simulink model "ammclib_gflib_pip_s32k14x"  (Simulink 9.0)
settings: Solver=FixedStepDiscrete  StartTime=0.0  StopTime=5  FixedStep=0.001  RelTol=1e-3  EnableMultiTasking=on
InitFcn:
  | mbd_s32k_consistency_checks(bdroot(gcs));
undefined symbols (not defined in the file or in its folder): LQFP
libraries: ammclib_bam_s32k14x x12, mbd_s32k1xx_ec_toolbox x2, simulink x1
Description:
  | This model tests the AMMCLIB GFLIB PI Parallel Form Controller blocks
  | 
  | Validation:
  | - Run the model in Simulation and check if the results look like the ones shown in the scope capture
  | - Open Freemaster (ammclib_gflib_pip_s32k14x.pmp) and compare the HW results against the Simulated ones
CloseFcn:
  | clear all;
settings Model: Creator=NXP MBDT Team  LastModifiedBy=nxf35172
settings DataIOCC: ExternalInput=off  InitialState=off  LimitDataPoints=on  SaveOutput=off  SignalLogging=off  SaveTime=off
settings OptimizationCC: DefaultParameterBehavior=Inlined  LifeSpan=1
settings DebuggingCC: SolverPrmCheckMsg=warning  InheritedTsInSrcMsg=none  SingleTaskRateTransMsg=error  ParameterPrecisionLossMsg=none  UnconnectedInputMsg=error  UnconnectedOutputMsg=error  UnconnectedLineMsg=error  AllowSymbolicDim=off  UnknownTsInhSupMsg=error  StateNameClashWarn=warning
settings HardwareCC: ProdLargestAtomicInteger=Long  ProdLargestAtomicFloat=Double  ProdEndianess=LittleEndian  ProdHWDeviceType=ARM Compatible->ARM Cortex
settings SFSimCC: MATLABDynamicMemAlloc=off
settings RTWCC: SystemTargetFile=mbd_s32k.tlc  MakeCommand=mbd_s32k_make_rtw COPY_MDLREF_INCLUDES=0  TemplateMakefile=mbd_s32k.tmf  Description=Model Based Design Toolbox S32K14x Code Generation Target
settings CodeAppCC: IgnoreCustomStorageClasses=off
settings STFCustomTargetCC: CombineOutputUpdateFcns=on  ERTCustomFileBanners=on  SupportContinuousTime=off  SupportNonInlinedSFcns=off  RemoveResetFunc=on  MATLABClassNameForMDSCustomization=Simulink.SoftwareTarget.ERTCustomization  GRTInterface=off  SystemTargetFile=mbd_s32k14.tlc
settings ERTTargetCC: MultiwordLength=2048  ParMdlRefBuildCompliant=off  CompOptLevelCompliant=off  ConcurrentExecutionCompliant=off  ModelStepFunctionPrototypeControlCompliant=off  CPPClassGenCompliant=off  UseToolchainInfoCompliant=off  InlinedParameterPlacement=NonHierarchical  ERTCustomFileTemplate=example_file_process.tlc  ConvertIfToSwitch=off  SuppressUnreachableDefaultCases=off  MaxIdInt32=FIRX_int32_T  MaxIdUint32=FIRX_uint32_T  MaxIdInt16=FIRX_int16_T  MaxIdUint16=FIRX_uint16_T  MaxIdInt8=FIRX_int8_T  MaxIdUint8=FIRX_uint8_T

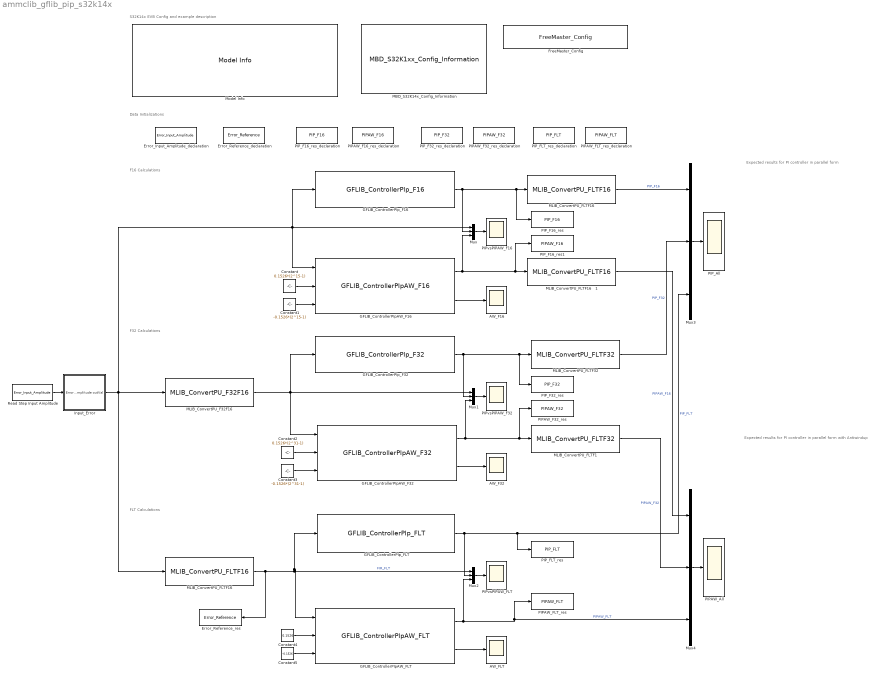
== system ammclib_gflib_pip_s32k14x ==
  note: Expected results for PI controller in parallel form with Antiwindup
  note: S32K14x EVB Config and example description
  note: Data Initializations
  note: F16 Calculations
  note: F32 Calculations
  note: FLT Calculations
  note: Expected results for PI controller in parallel form
  AW_F16 : Scope
  AW_F32 : Scope
  AW_FLT : Scope
  Constant : Constant  Value=0.1526*(2^15-1)  OutDataTypeStr=Inherit: Inherit via back propagation
  Constant1 : Constant  Value=-0.1526*(2^15-1)  OutDataTypeStr=Inherit: Inherit via back propagation
  Constant2 : Constant  Value=0.1526*(2^31-1)  OutDataTypeStr=Inherit: Inherit via back propagation
  Constant3 : Constant  Value=-0.1526*(2^31-1)  OutDataTypeStr=Inherit: Inherit via back propagation
  Constant4 : Constant  Value=0.1526  OutDataTypeStr=Inherit: Inherit via back propagation
  Constant5 : Constant  Value=-0.1526  OutDataTypeStr=Inherit: Inherit via back propagation
  Error_Input_Amplitude_declaration : DataStoreMemory  Priority=1  DataStoreName=Error_Input_Amplitude  WriteAfterWriteMsg=warning  WriteAfterReadMsg=warning  InitialValue=8192  ShowAdditionalParam=off  OutMin=-32768  OutMax=32767  OutDataTypeStr=int16
  Error_Reference_declaration : DataStoreMemory  Priority=1  DataStoreName=Error_Reference  WriteAfterWriteMsg=warning  WriteAfterReadMsg=warning  ShowAdditionalParam=off  OutMin=-1  OutMax=1  OutDataTypeStr=single
  Error_Reference_res : DataStoreWrite  DataStoreName=Error_Reference
  FreeMaster_Config : mbd_s32k1xx_ec_toolbox/Utility Blocks/FreeMaster_Config  interface=LPUART1  baudrate=115200  rxd=PTC6: [LPUART1_RX | Receive]  txd=PTC7: [LPUART1_TX | Transmit]  mode=Short Interrupt  isr_prio=15  show_adv_opts=off  use_scope=on  max_scope_vars=8  use_recorder=on  max_rec_vars=8  rec_buff_size=1024  rec_timebase=0 milliseconds  comm_buffer_size_auto=on  comm_buffer_size=255  comm_rqueue_size_default=on  comm_rqueue_size=32
  GFLIB_ControllerPIpAW_F16 : ammclib_bam_s32k14x/GFLIB/bam_f16/GFLIB_ControllerPIpAW_F16  f16PropGain=0.006*(2^15-1)  s16PropGainShift=0  f16IntegGain=0.0006*(2^15-1)  s16IntegGainShift=0
  GFLIB_ControllerPIpAW_F32 : ammclib_bam_s32k14x/GFLIB/bam_f32/GFLIB_ControllerPIpAW_F32  f32PropGain=0.006*(2^31-1)  s16PropGainShift=0  f32IntegGain=0.0006*(2^31-1)  s16IntegGainShift=0
  GFLIB_ControllerPIpAW_FLT : ammclib_bam_s32k14x/GFLIB/bam_flt/GFLIB_ControllerPIpAW_FLT  fltPropGain=0.006  fltIntegGain=0.0006
  GFLIB_ControllerPIp_F16 : ammclib_bam_s32k14x/GFLIB/bam_f16/GFLIB_ControllerPIp_F16  f16PropGain=0.006*(2^15-1)  s16PropGainShift=0  f16IntegGain=0.0006*(2^15-1)  s16IntegGainShift=0
  GFLIB_ControllerPIp_F32 : ammclib_bam_s32k14x/GFLIB/bam_f32/GFLIB_ControllerPIp_F32  f32PropGain=0.006*(2^31-1)  s16PropGainShift=0  f32IntegGain=0.0006*(2^31-1)  s16IntegGainShift=0
  GFLIB_ControllerPIp_FLT : ammclib_bam_s32k14x/GFLIB/bam_flt/GFLIB_ControllerPIp_FLT  fltPropGain=0.006  fltIntegGain=0.0006
  Input_Error : Stateflow chart  TreatAsAtomicUnit=on
  MBD_S32K14x_Config_Information : mbd_s32k1xx_ec_toolbox/MBD_S32K1xx_Config_Information  Priority=0  mbdt_ver=0  disp_str=|  config_params=[]  mcu_target_name=S32K144  mcu_target_package=100-LQFP  mcu_target_sram_size=64KB  mcu_system_clock_freq=80  mcu_xtal_freq=External 8  mcu_steptick_timer=LPIT Channel 0  mcu_steptick_prio=15  ds_import_enable=on  target_compiler=GCC  target_memory=FLASH  gcc_target_compile_opts=-mcpu=cortex-m4 -mthumb -mfloat-abi=hard -mfpu=fpv4-sp-d16 -O1 -g -gstrict-dwarf  gcc_target_assemble_opts=-mcpu=cortex-m4 -mthumb -mfloat-abi=hard -mfpu=fpv4-sp-d16 -g  gcc_target_link_opts=-mcpu=cortex-m4 -mthumb -mfloat-abi=hard -mfpu=fpv4-sp-d16  gcc_target_default_lcf=on  gcc_target_user_lcf=S32K144_64_flash.ld  ghs_target_compile_opts=-cpu=cortexm4f -thumb -DARM_MATH_CM4 -fpu=vfpv4_d16 -fsingle -Ogeneral -Wundef -Wimplicit-int -Wshadow -Wtrigraphs --no_commons --gnu_asm -gnu99 -gdwarf-2 -G  ghs_target_assemble_opts=-cpu=cortexm4f -fpu=vfpv4_d16  ghs_target_link_opts=-cpu=cortexm4f -thumb -fpu=vfpv4_d16  ghs_target_default_lcf=off  ghs_target_user_lcf=S32K144_64_flash.ld  iar_target_compile_opts=--cpu=Cortex-M4F --thumb --fpu=VFPv4_sp -Ol -e --debug --dlib_config normal  iar_target_assemble_opts=--cpu Cortex-M4F --thumb --fpu VFPv4_sp  iar_target_link_opts=--no_exceptions --vfe --inline  iar_target_default_lcf=off  iar_target_user_lcf=S32K144_64_flash.icf  pil_download_enable=off  rbl_download_enable=on  rbl_start_delay=5000000  rbl_download_interface=OpenSDA  rbl_restart_request=off  rbl_com_port=Custom  rbl_com_port_custom=COM1  pil_download_rate=57600  pil_opensda_drive=Custom  pil_opensda_drive_custom=D  pil_uart_instance=0  pil_uart_rx=PTA2: [LPUART0_RX | Receive]  pil_uart_tx=PTA3: [LPUART0_TX | Transmit]  FTM_PWM_PcrCheckEnDis=on  FTM_Input_Edge_Inputs_PcrCheckEnDis=on  FTM_Dual_Edge_Inputs_PcrCheckEnDis=on  FTM_Quadrature_Inputs_PcrCheckEnDis=on  FTM_Hall_Sensor_Inputs_PcrCheckEnDis=on  LPTMR_PcrCheckEnDis=on  PIT_PcrCheckEnDis=on  RTC_PcrCheckEnDis=on  FlexCAN_PcrCheckEnDis=on  LIN_PcrCheckEnDis=on  FlexIO_PcrCheckEnDis=on  LPI2C_PcrCheckEnDis=on  LPSPI_PcrCheckEnDis=on  LPUART_PcrCheckEnDis=on  CMP_PcrCheckEnDis=on  GPIO_OutputPcrCheckEnDis=on  GPIO_InputPcrCheckEnDis=on  SBC_PcrCheckEnDis=on  AMMCLIB_PcrCheckEnDis=on  FM_PcrCheckEnDis=on  Profile_PcrCheckEnDis=on  ConfigParams_PcrCheckEnDis=on  ModelRef_PcrCheckEnDis=on  PDB0_PcrCheckEnDis=on  CSEc_PcrCheckEnDis=on  eDMA_PcrCheckEnDis=on  ADC_PcrCheckEnDis=on  WDOG_PcrCheckEnDis=on
      | Target : S32K142-16KB_SRAM
      | Package : 100-pin
      | System clock : 80 MHz
      | XTAL clock : External 8 MHz
      | Compiler : GCC
      | Target Type : FLASH
      | Download Code after build : (OpenSDA: E)
      | Step Tick Interrupt Priority : 15
  MLIB_ConvertPU_F32F16 : ammclib_bam_s32k14x/MLIB/bam_f32/MLIB_ConvertPU_F32F16
  MLIB_ConvertPU_FLTF1 : ammclib_bam_s32k14x/MLIB/bam_flt/MLIB_ConvertPU_FLTF32
  MLIB_ConvertPU_FLTF16 : ammclib_bam_s32k14x/MLIB/bam_flt/MLIB_ConvertPU_FLTF16
  "MLIB_ConvertPU_FLTF16   " : ammclib_bam_s32k14x/MLIB/bam_flt/MLIB_ConvertPU_FLTF16
  MLIB_ConvertPU_FLTF16   1 : ammclib_bam_s32k14x/MLIB/bam_flt/MLIB_ConvertPU_FLTF16
  MLIB_ConvertPU_FLTF32 : ammclib_bam_s32k14x/MLIB/bam_flt/MLIB_ConvertPU_FLTF32
  Model Info : simulink/Model-Wide Utilities/Model Info  Frame=off  DisplayStringWithTags=|  HorizontalTextAlignment=Left  LeftAlignmentValue=0.02
      | Model Name: %<ModelName>
      | 
      | Description: %<Description>
  Mux{,1..4} (5 alike) : Mux  Inputs=3
  PIPAW_All : Scope
  PIPAW_F16_res_declaration : DataStoreMemory  Priority=2  DataStoreName=PIPAW_F16  ReadBeforeWriteMsg=warning  WriteAfterWriteMsg=warning  WriteAfterReadMsg=warning  ShowAdditionalParam=off  OutDataTypeStr=int16
  PIPAW_F32_res : DataStoreWrite  DataStoreName=PIPAW_F32
  PIPAW_F32_res_declaration : DataStoreMemory  Priority=2  DataStoreName=PIPAW_F32  ReadBeforeWriteMsg=warning  WriteAfterWriteMsg=warning  WriteAfterReadMsg=warning  ShowAdditionalParam=off  OutDataTypeStr=int32
  PIPAW_FLT_res : DataStoreWrite  DataStoreName=PIPAW_FLT
  PIPAW_FLT_res_declaration : DataStoreMemory  Priority=2  DataStoreName=PIPAW_FLT  ReadBeforeWriteMsg=warning  WriteAfterWriteMsg=warning  WriteAfterReadMsg=warning  ShowAdditionalParam=off  OutDataTypeStr=single
  PIP_All : Scope
  PIP_F16_res : DataStoreWrite  DataStoreName=PIP_F16
  PIP_F16_res1 : DataStoreWrite  DataStoreName=PIPAW_F16
  PIP_F16_res_declaration : DataStoreMemory  Priority=2  DataStoreName=PIP_F16  ReadBeforeWriteMsg=warning  WriteAfterWriteMsg=warning  WriteAfterReadMsg=warning  ShowAdditionalParam=off  OutDataTypeStr=int16
  PIP_F32_res : DataStoreWrite  DataStoreName=PIP_F32
  PIP_F32_res_declaration : DataStoreMemory  Priority=2  DataStoreName=PIP_F32  ReadBeforeWriteMsg=warning  WriteAfterWriteMsg=warning  WriteAfterReadMsg=warning  ShowAdditionalParam=off  OutDataTypeStr=int32
  PIP_FLT_res : DataStoreWrite  DataStoreName=PIP_FLT
  PIP_FLT_res_declaration : DataStoreMemory  Priority=2  DataStoreName=PIP_FLT  ReadBeforeWriteMsg=warning  WriteAfterWriteMsg=warning  WriteAfterReadMsg=warning  ShowAdditionalParam=off  OutDataTypeStr=single
  PIPvsPIPAW_F16 : Scope
  PIPvsPIPAW_F32 : Scope
  PIPvsPIPAW_FLT : Scope
  Read Step Input Amplitude : DataStoreRead  DataStoreName=Error_Input_Amplitude
  wires:
  Input_Error/1(outVal) -> GFLIB_ControllerPIp_F16/1, GFLIB_ControllerPIpAW_F16/1, Mux/1, MLIB_ConvertPU_FLTF16/1, MLIB_ConvertPU_F32F16/1
  GFLIB_ControllerPIp_F16/1 -> "MLIB_ConvertPU_FLTF16   "/1, PIP_F16_res/1, Mux/2
  Mux/1 -> PIPvsPIPAW_F16/1
  Read Step Input Amplitude/1 -> Input_Error/1(Error_Input_Amplitude)
  MLIB_ConvertPU_FLTF16/1 -> Error_Reference_res/1, GFLIB_ControllerPIp_FLT/1, GFLIB_ControllerPIpAW_FLT/1, Mux2/1  "FIR_FLT"
  Constant/1 -> GFLIB_ControllerPIpAW_F16/2
  Constant1/1 -> GFLIB_ControllerPIpAW_F16/3
  GFLIB_ControllerPIpAW_F16/2 -> AW_F16/1
  GFLIB_ControllerPIpAW_F16/1 -> PIP_F16_res1/1, MLIB_ConvertPU_FLTF16   1/1, Mux/3
  "MLIB_ConvertPU_FLTF16   "/1 -> Mux3/1  "PIP_F16"
  MLIB_ConvertPU_FLTF16   1/1 -> Mux4/1  "PIPAW_F16"
  GFLIB_ControllerPIp_F32/1 -> Mux1/2, MLIB_ConvertPU_FLTF32/1, PIP_F32_res/1
  GFLIB_ControllerPIpAW_F32/1 -> Mux1/3, PIPAW_F32_res/1, MLIB_ConvertPU_FLTF1/1
  Mux1/1 -> PIPvsPIPAW_F32/1
  MLIB_ConvertPU_F32F16/1 -> GFLIB_ControllerPIpAW_F32/1, Mux1/1, GFLIB_ControllerPIp_F32/1
  GFLIB_ControllerPIpAW_F32/2 -> AW_F32/1
  Constant2/1 -> GFLIB_ControllerPIpAW_F32/2
  Constant3/1 -> GFLIB_ControllerPIpAW_F32/3
  MLIB_ConvertPU_FLTF32/1 -> Mux3/2  "PIP_F32"
  MLIB_ConvertPU_FLTF1/1 -> Mux4/2  "PIPAW_F32"
  GFLIB_ControllerPIp_FLT/1 -> Mux2/2, Mux3/3, PIP_FLT_res/1  "PIP_FLT"
  Mux2/1 -> PIPvsPIPAW_FLT/1
  GFLIB_ControllerPIpAW_FLT/1 -> Mux4/3, PIPAW_FLT_res/1, Mux2/3  "PIPAW_FLT"
  GFLIB_ControllerPIpAW_FLT/2 -> AW_FLT/1
  Constant5/1 -> GFLIB_ControllerPIpAW_FLT/3
  Constant4/1 -> GFLIB_ControllerPIpAW_FLT/2
  Mux3/1 -> PIP_All/1
  Mux4/1 -> PIPAW_All/1

== stateflow chart Input_Error ==
  settings: executeAtInitialization=1
  state A
    du:
    outVal = Error_Input_Amplitude;
    cntr=cntr+1;
  state A1
    du:
    outVal = -Error_Input_Amplitude;
    cntr=cntr-1;
  (default) -> A : {cntr=0;}
  A1 -> A : [cntr < 2]
  A -> A1 : [cntr > 1000]
  data: cntr local uint32 [0..12] =0; outVal output int16; Error_Input_Amplitude input int16
